simulink model "ModeloManual"  (R2022a)
settings: Solver=VariableStepAuto  StartTime=0.0  StopTime=10  RelTol=1e-3
values from neighbouring files (symbols this model uses):
  a = 0.2    [Data.m]
  alturaobst = 0.9    [Data.m]
  b = 0.542    [Data.m]
  M = [x_new y_new]    [Data.m]
  M_chasis = 3    [Data.m]
  M_rueda = 1    [Data.m]
  M_ruedacontacto = 1    [Data.m]
  N = 4365    [GraficasVelocidades.m]    (also in Prueba_Liapunov.m = length(p_X); WaypointsToTrayectory.m = length(X))
  R = 0.175/2    (= 0.0875)    [Data.m]
  X = M(:,1)    [WaypointsToTrayectory.m]
  x0 = x_ini(1)*factorE    [Data.m]
  x_obj = pos_fin(1)*factorE    [Data.m]
  xobstac = RandomPos(1)    [Data.m]
  Y = M(:, 2)    [WaypointsToTrayectory.m]
  y0 = y_ini(2)*factorE    [Data.m]
  y_obj = pos_fin(2)*factorE    [Data.m]
  yobstac = RandomPos(2)    [Data.m]
  zobstac = RandomPos(3)    [Data.m]
undefined symbols (not defined in the file or in its folder): bloqueobstaculo, Borde11, Borde12, Borde2, Borde3, Borde41, Borde42, Explanada, plano150g1, plano150g2, plano150g3, plano150g4, Plano150mm, plano150mm2irr, Plano45mm, plano45mm2irr, Plano90mm, Rampa, Rampa21, Rampa22, Rampa31, Rampa32, Rampa33, Rampa4, Rampa51, Rampa52, Rampa53, Terreno, Z
libraries: sm_lib x331, nesl_utility x30, fl_lib x3, robotalgslib x1
(part 1 of 8)
settings Model: Creator=User  LastModifiedBy=User
settings ExplorerConfigSet: InternalSimMechanicsExplorerSettings="<ExplorerConfiguration><canonicalview>default</canonicalview><AnimationSetting><BasePlaybackSpeed>1.0</BasePlaybackSpeed><PlaybackSpeedFactor>8.0</PlaybackSpeedFactor></AnimationSetting><TilePanel><TileInfo><Tiles Columns=\"2\" Count=\"2\" Rows=\"1\"><Column Weight=\"0.5166\"/><Column Weight=\"0.4834\"/><Row Weight=\"1\"/><Tile Height=\"1\" Width=\"1\" X=\"0\" Y=\"0\"/><Tile Height=\"1\" Width=\"1\" X=\"1\" Y=\"0\"/></Tiles></TileInfo><SceneInfo><SceneViewer><BGColor><R>0.60000002384185791</R><G>0.60000002384185791</G><B>0.60000002384185791</B></BGColor><Camera><DoPerspective>on</DoPerspective><Position><X>190.872114263138826</X><Y>194.191955454598997</Y><Z>244.498723214842585</Z></Position><Center><X>176.122953180660318</X><Y>239.114971855998164</Y><Z>2.09998758117879447</Z></Center><Up><X>0.0154631214745943289</X><Y>0.983307639935577793</Y><Z>0.181292518098750938</Z></Up><ViewLimDist>1</ViewLimDist><YLim>0.466307658154998583</YLim><XLim>0.450624665167722871</XLim></Camera></SceneViewer><SceneViewer><BGColor><R>0.400000005960464478</R><G>0.800000011920928955</G><B>1</B></BGColor><Camera><DoPerspective>on</DoPerspective><Position><X>214.286586538195536</X><Y>301.219122430627294</Y><Z>1.50750834751243712</Z></Position><Center><X>214.645296115876107</X><Y>302.136282732512313</Y><Z>1.33388686403077461</Z></Center><Up><X>0.0632456935347918969</X><Y>0.16169230597039197</Y><Z>0.984812459526828055</Z></Up><ViewLimDist>1</ViewLimDist><YLim>0.466307658154998583</YLim><XLim>0.421349744924808145</XLim></Camera></SceneViewer></SceneInfo></TilePanel><MechEditorPanel><Cameras><Camera><Id>Camera2</Id><Value><Name>Seguimiento</Name><NativeCamera><PositionTrackingFeature>ROBOT_SS.Ensamble_robot.Chasis.Chasis_Camera_RightB.R</PositionTrackingFeature><CenterTrackingFeature>ROBOT_SS.Ensamble_robot.Chasis.Chasis_Camera_RightB.R</CenterTrackingFeature><UpVectorTrackingFeature>ROBOT_SS.Ensamble_robot.Chasis.Chasis_Camera_RightB.R</UpVectorTrackingFeature><CenterTrackingOrigin>off</CenterTrackingOrigin><CenterTrackingDirection>+X</CenterTrackingDirection><UpVectorTrackingDirection>+Z</UpVectorTrackingDirection></NativeCamera></Value></Camera><Camera><Id>Camera3</Id><Value><Name>Fija</Name><NativeCamera><PositionKeyframeSet><Keyframe><Time>10</Time><Value><X>194.17156367953794</X><Y>236.62255003194693</Y><Z>376.38019149049347</Z></Value></Keyframe></PositionKeyframeSet><CenterKeyframeSet><Keyframe><Time>10</Time><Value><X>194.17156367953794</X><Y>236.62255003194693</Y><Z>15.721481323242188</Z></Value></Keyframe></CenterKeyframeSet><UpVectorKeyframeSet><Keyframe><Time>10</Time><Value><X>0</X><Y>1</Y><Z>-0</Z></Value></Keyframe></UpVectorKeyframeSet></NativeCamera></Value></Camera><Camera><Id>Camera4</Id><Value><Name>lateralVista</Name><NativeCamera><PositionTrackingFeature>ROBOT_SS.Ensamble_robot.Chasis.Chasis_Camera_Rear.R</PositionTrackingFeature><CenterTrackingFeature>ROBOT_SS.Ensamble_robot.Chasis.Chasis_Camera_Rear.R</CenterTrackingFeature><UpVectorTrackingFeature>ROBOT_SS.Ensamble_robot.Chasis.Chasis_Camera_Rear.R</UpVectorTrackingFeature><CenterTrackingOrigin>off</CenterTrackingOrigin><CenterTrackingDirection>-Y</CenterTrackingDirection><UpVectorTrackingDirection>+Z</UpVectorTrackingDirection></NativeCamera></Value></Camera><Camera><Id>Camera5</Id><Value><Name>VistaAsup</Name><NativeCamera><PositionTrackingFeature>ROBOT_SS.Ensamble_robot.Chasis.Chasis_Camera_RightA.R</PositionTrackingFeature><CenterTrackingFeature>ROBOT_SS.Ensamble_robot.Chasis.Chasis_Camera_RightA.R</CenterTrackingFeature><UpVectorTrackingFeature>ROBOT_SS.Ensamble_robot.Chasis.Chasis_Camera_RightA.R</UpVectorTrackingFeature><CenterTrackingOrigin>off</CenterTrackingOrigin><CenterTrackingDirection>+X</CenterTrackingDirection><UpVectorTrackingDirection>+Z</UpVectorTrackingDirection></NativeCamera></Value></Camera><Camera><Id>Camera6</Id><Value><Name>VistaB</Name><NativeCamera><PositionTrackingFeature>ROBOT_SS.Ensamble_robot.Chasis.Chasis_Camera_RightB.R</PositionTrackingFeature><CenterTrackingFeature>ROBOT_SS.Ensamble_robot.Chasis.Chasis_Camera_RightB.R</CenterTrackingFeature><UpVectorTrackingFeature>ROBOT_SS.Ensamble_robot.Chasis.Chasis_Camera_RightB.R</UpVectorTrackingFeature><CenterTrackingOrigin>off</CenterTrackingOrigin><CenterTrackingDirection>+X</CenterTrackingDirection><UpVectorTrackingDirection>+Z</UpVectorTrackingDirection></NativeCamera></Value></Camera><Camera><Id>Camera7</Id><Value><Name>Top</Name><NativeCamera><PositionKeyframeSet><Keyframe><Time>0</Time><Value><X>190.87211426313883</X><Y>194.191955454599</Y><Z>244.49872321484258</Z></Value></Keyframe></PositionKeyframeSet><CenterKeyframeSet><Keyframe><Time>0</Time><Value><X>176.12295318066032</X><Y>239.11497185599816</Y><Z>2.0999875811787945</Z></Value></Keyframe></CenterKeyframeSet><UpVectorKeyframeSet><Keyframe><Time>0</Time><Value><X>0.015463121474594329</X><Y>0.98330763993557779</Y><Z>0.18129251809875094</Z></Value></Keyframe></UpVectorKeyframeSet></NativeCamera></Value></Camera></Cameras><GfxPanelCameraMap><MapElement CameraMLId=\"Camera7\" GfxPanelIndex=\"0\"/><MapElement CameraMLId=\"Camera5\" GfxPanelIndex=\"1\"/></GfxPanelCameraMap><VideoCreator><PlaybackSpeedRatio>4.0</PlaybackSpeedRatio><FrameRate>60</FrameRate><VideoFormat>MPEG-4</VideoFormat><FrameSize>auto</FrameSize></VideoCreator></MechEditorPanel></ExplorerConfiguration>"

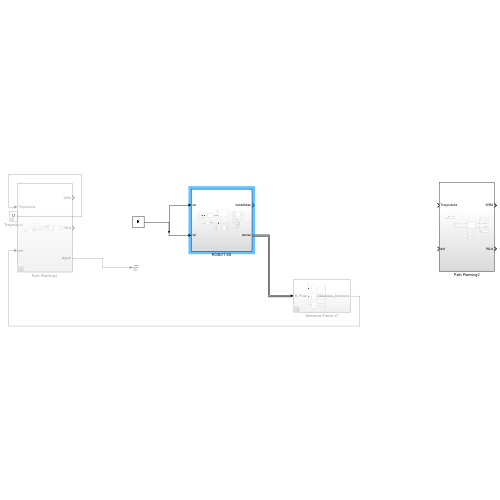
[thumbnail: Simulink's stored preview of the top-level diagram]
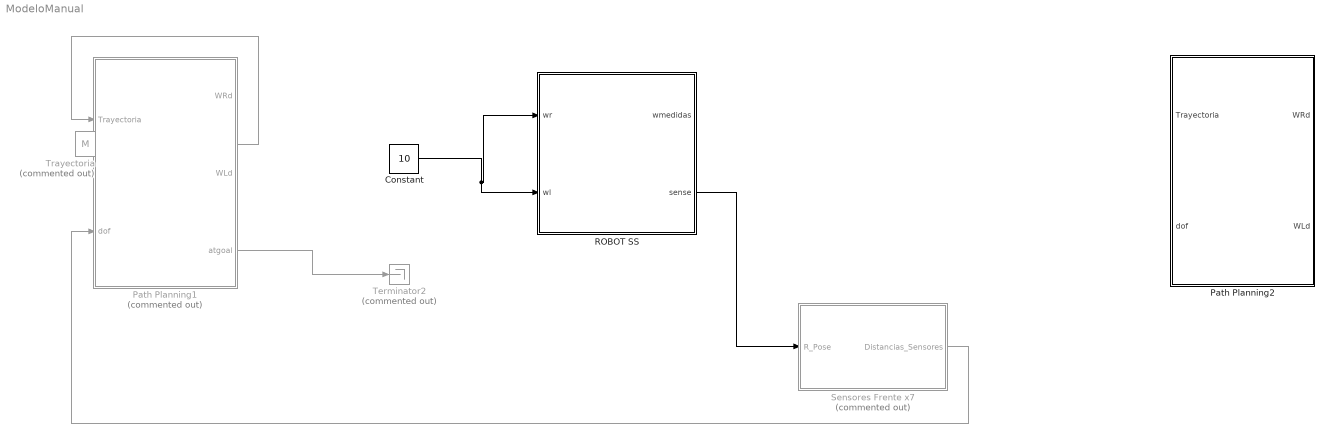
== system ModeloManual ==
  Constant : Constant  Value=10
  Path Planning1 : Subsystem  Commented=on
  Path Planning2 : Subsystem
  ROBOT SS : Subsystem
  Sensores Frente x7 : Subsystem  Commented=on
  Terminator2 : Terminator  Commented=on
  Trayectoria : Constant  Commented=on  Value=M
  wires:
  Path Planning1/3(atgoal) -> Terminator2/1
  Trayectoria/1 -> Path Planning1/1(Trayectoria)
  ROBOT SS/2(sense) -> Sensores Frente x7/1(R_Pose)
  Constant/1 -> ROBOT SS/2(wl), ROBOT SS/1(wr)
  Sensores Frente x7/1(Distancias_Sensores) -> Path Planning1/2(dof)

== system ModeloManual/Path Planning1 ==
  note: Des Wspeed
  Trayectoria : Inport
  In Bus Element : Inport  Port=2  PortName=dof  Element=Pose
  Clock : Clock
  Constant : Constant  Value=0.5
  Kinematics1 : Subsystem
  Pure  Pursuit2 : robotalgslib/Pure Pursuit  DesiredLinearVelocity=1.38  MaxAngularVelocity=pi  LookaheadDistance=0.05  TargetDirPort=on  SimulateUsing=Interpreted execution
  Subsystem1 : Subsystem
  Terminator : Terminator
  Terminator1 : Terminator
  To Workspace : ToWorkspace  VariableName=RobotPose  SampleTime=-1
  Trapezoidal Vel Profile : MATLAB Function  TreatAsAtomicUnit=on
  hold : Subsystem
  t1 : Constant
  WRd : Outport
  WLd : Outport  Port=2
  atgoal : Outport  Port=3
  wires:
  Pure  Pursuit2/1 -> Trapezoidal Vel Profile/1(linVel), Subsystem1/1(linearV)
  Constant/1 -> Trapezoidal Vel Profile/4(accel)
  Clock/1 -> Trapezoidal Vel Profile/2(t)
  Kinematics1/1(WRd) -> WRd/1
  Pure  Pursuit2/2 -> Kinematics1/2(w)
  Trapezoidal Vel Profile/1(lin_Vel_out) -> Kinematics1/1(v)
  t1/1 -> Trapezoidal Vel Profile/3(t1)
  hold/1(deaccelStartTime) -> Trapezoidal Vel Profile/5(deaccelStartTime)
  Trayectoria/1 -> Pure  Pursuit2/2
  Subsystem1/2(atgoal) -> atgoal/1
  Subsystem1/1(deAcc) -> hold/1(deAcc)
  Kinematics1/2(WLd) -> WLd/1
  In Bus Element/1 -> Subsystem1/2(Pose), To Workspace/1, Pure  Pursuit2/1
  Pure  Pursuit2/3 -> Terminator/1
  Kinematics1/3(Pose) -> Terminator1/1

== system ModeloManual/Path Planning2 ==
  Trayectoria : Inport
  In Bus Element : Inport  Port=2  PortName=dof  Element=Pose
  Constant : Constant  Value=1.38
  Constant1 : Constant  Value=0
  Display{,1..3} (4 alike) : Display
  Kinematics1 : Subsystem
  Waypoint Tracking Logic : Stateflow chart  Commented=on  TreatAsAtomicUnit=on
  WRd : Outport
  WLd : Outport  Port=2
  wires:
  Constant1/1 -> Kinematics1/2(w)
  Constant/1 -> Kinematics1/1(v)
  Trayectoria/1 -> Waypoint Tracking Logic/2(waypoints)
  In Bus Element/1 -> Waypoint Tracking Logic/1(pose)
  Kinematics1/2(WLd) -> WLd/1, Display3/1
  Kinematics1/1(WRd) -> Display1/1, WRd/1

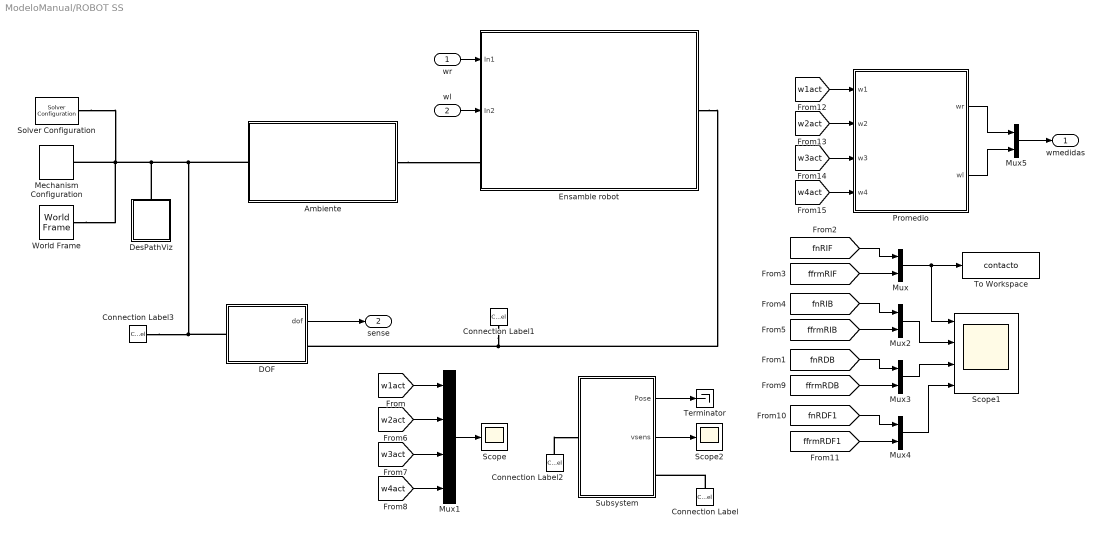
== system ModeloManual/ROBOT SS ==
  wr : Inport
  wl : Inport  Port=2
  Ambiente : Subsystem
  Connection Label : ConnectionLabel  Label=Ref
  Connection Label1 : ConnectionLabel  Label=Ref
  Connection Label2 : ConnectionLabel  Label=B
  Connection Label3 : ConnectionLabel  Label=B
  DOF : Subsystem
  DesPathViz : Subsystem
  Ensamble robot : Subsystem
  Mechanism Configuration : sm_lib/Utilities/Mechanism Configuration  UniformGravity=Constant  GravityVector=[0 0 -9.80665]  GravityUnits=m/s^2  LinearizationDelta=0.001  JointModeTransitionNonlinearIterations=2
  Mux{,2..5} (5 alike) : Mux  Inputs=2
  Mux1 : Mux
  Promedio : MATLAB Function  TreatAsAtomicUnit=on
  Scope : Scope
  Scope1 : Scope  NumInputPorts=4
  Scope2 : Scope
  Solver Configuration : nesl_utility/Solver Configuration  PhysicalDomain=network_engine_domain  SubClassName=solver  LeftPortType=input  RightPortType=generic  Tones=[]  Harmonics=[]  SimulateNoise=off  Profile=off  UseLocalSampling=off  EnableSwitchedLinearOptims=on  FrequencyDomain=off  UseCCode=off  RelTol=0.001  AbsTol=0.001  MinStep=1e-09  ToWorkspace=off  RevertToSquareIcSolve=off  NumHomotopyIterations=100  PhasorMode=off  PhasorModeNumHarmonics=1  IndexReductionMethod=DerivativeReplacement  DoDC=off  ResidualTolerance=1e-09  UseLocalSolver=off  LocalSolverChoice=NE_BACKWARD_EULER_ADVANCER  LocalSolverSampleTime=0.001  DoFixedCost=off  MaxNonlinIter=3  MaxModeIter=2  ComputeImpulses=off  ImpulseIterations=2  LinearAlgebra=auto  LinearAlgebraNumThread=0  EquationFormulation=NE_TIME_EF  DelaysMemoryBudget=1024  AutomaticFiltering=on  FilteringTimeConstant=0.001  PartitionStorageMethod=AS_NEEDED  PartitionMemoryBudget=1024  PartitionMethod=ROBUST
      settings: SourceProductBaseCode=SS,PW,VE
  Subsystem : Subsystem
  Terminator : Terminator
  To Workspace : ToWorkspace  VariableName=contacto  SaveFormat=Timeseries  SampleTime=-1
  World Frame : sm_lib/Frames and Transforms/World Frame
  wmedidas : Outport
  sense : Outport  Port=2
  wires:
  [w3act] -> Mux1/3
  [w1act] -> Mux1/1
  Mux1/1 -> Scope/1
  [w2act] -> Mux1/2
  [w4act] -> Mux1/4
  [ffrmRDB] -> Mux3/2
  Mux/1 -> Scope1/1, To Workspace/1
  [ffrmRIF] -> Mux/2
  [ffrmRIB] -> Mux2/2
  [fnRDB] -> Mux3/1
  Mux3/1 -> Scope1/3
  [fnRIF] -> Mux/1
  Mux2/1 -> Scope1/2
  Mux4/1 -> Scope1/4
  [fnRDF1] -> Mux4/1
  [fnRIB] -> Mux2/1
  [ffrmRDF1] -> Mux4/2
  Mux5/1 -> wmedidas/1
  [w3act] -> Promedio/3(w3)
  [w4act] -> Promedio/4(w4)
  [w1act] -> Promedio/1(w1)
  Promedio/2(wl) -> Mux5/2
  [w2act] -> Promedio/2(w2)
  Promedio/1(wr) -> Mux5/1
  DOF/1(dof) -> sense/1
  Subsystem/2(vsens) -> Scope2/1
  Subsystem/1(Pose) -> Terminator/1
  wr/1 -> Ensamble robot/1(In1)
  wl/1 -> Ensamble robot/2(In2)
  connections:
  Connection Label/LConn1 -- Subsystem/RConn1
  Connection Label2/LConn1 -- Subsystem/LConn1
  Ensamble robot/RConn1 -- DOF/RConn1 -- Connection Label1/LConn1
  Ambiente/RConn1 -- Ensamble robot/LConn1
  DOF/LConn1 -- Ambiente/LConn1 -- Solver Configuration/RConn1 -- Mechanism Configuration/RConn1 -- World Frame/RConn1 -- DesPathViz/LConn1 -- Connection Label3/LConn1

== system ModeloManual/Sensores Frente x7 ==
  R_Pose : Inport
  Mux : Mux  Inputs=7
  Percepción_Central : Subsystem
  Percepción_Derecha : Subsystem
  Percepción_Izquierda : Subsystem
  Distancias_Sensores : Outport
  wires:
  Percepción_Derecha/2(d_7) -> Mux/7
  Percepción_Central/2(d_4) -> Mux/4
  Percepción_Derecha/1(d_6) -> Mux/6
  Percepción_Izquierda/2(d_2) -> Mux/2
  Percepción_Central/1(d_3) -> Mux/3
  R_Pose/1 -> Percepción_Izquierda/1(R_Pose), Percepción_Central/1(R_Pose), Percepción_Derecha/1(R_Pose)
  Percepción_Izquierda/1(d_1) -> Mux/1
  Percepción_Central/3(d_5) -> Mux/5
  Mux/1 -> Distancias_Sensores/1

== system ModeloManual/Path Planning1/Kinematics1 ==
  v : Inport
  w : Inport  Port=2
  Direct-Kinematics : Subsystem
  Inverse-Kinematics : Subsystem
  Scope1 : Scope  NumInputPorts=2
  WRd : Outport
  WLd : Outport  Port=2
  Pose : Outport  Port=3
  wires:
  Direct-Kinematics/1(Pose) -> Pose/1
  Inverse-Kinematics/1(wL) -> WLd/1, Direct-Kinematics/1(wl), Scope1/1
  Inverse-Kinematics/2(wR) -> WRd/1, Direct-Kinematics/2(wr), Scope1/2
  w/1 -> Direct-Kinematics/3(w), Inverse-Kinematics/2(w)
  v/1 -> Inverse-Kinematics/1(v)

== system ModeloManual/Path Planning1/Subsystem1 ==
  linearV : Inport
  Pose : Inport  Port=2
  Add : Sum
  Constant : Constant  Value=2* 0.5
  Constant1 : Constant  Value=0.25
  Gain : Gain
  GreaterThan : RelationalOperator  Operator=>  OutDataTypeStr=boolean  RndMeth=Simplest  InputSameDT=off
  GreaterThan1 : RelationalOperator  Operator=>  OutDataTypeStr=boolean  RndMeth=Simplest  InputSameDT=off
  NOT : Logic  Operator=NOT  IconShape=distinctive  AllPortsSameDT=off  OutDataTypeStr=boolean
  Product : Product  Inputs=*/
  Square : Math  Operator=square
  Unit Delay : UnitDelay  SampleTime=-1  HasFrameUpgradeWarning=on
  check-goal : Subsystem
  deAcc : Outport
  atgoal : Outport  Port=2
  wires:
  check-goal/1(distanceGoal) -> GreaterThan/1, GreaterThan1/1
  Constant/1 -> Product/2
  Constant1/1 -> GreaterThan1/2, Gain/1
  Add/1 -> GreaterThan/2
  Product/1 -> Add/1
  GreaterThan1/1 -> NOT/1
  Square/1 -> Product/1
  GreaterThan/1 -> deAcc/1
  NOT/1 -> Unit Delay/1
  Pose/1 -> check-goal/1(Pose)
  Unit Delay/1 -> atgoal/1
  linearV/1 -> Square/1
  Gain/1 -> Add/2

== system ModeloManual/Path Planning1/hold ==
  deAcc : Inport
  Constant9 : Constant  Value=inf
  NOT1 : Logic  Operator=NOT  IconShape=distinctive  AllPortsSameDT=off  OutDataTypeStr=boolean
  StopTime : Subsystem
  Switch3 : Switch  Criteria=u2 > Threshold  SaturateOnIntegerOverflow=off  InputSameDT=off
  Unit Delay1 : UnitDelay  SampleTime=-1  HasFrameUpgradeWarning=on
  deaccelStartTime : Outport
  wires:
  Unit Delay1/1 -> Switch3/2
  StopTime/1(DeAccelTime) -> Switch3/1
  Switch3/1 -> deaccelStartTime/1
  NOT1/1 -> StopTime/1(Enable), Unit Delay1/1
  Constant9/1 -> Switch3/3
  deAcc/1 -> NOT1/1

== system ModeloManual/Path Planning2/Kinematics1 ==
  v : Inport
  w : Inport  Port=2
  Inverse-Kinematics : Subsystem
  Scope1 : Scope  NumInputPorts=2
  WRd : Outport
  WLd : Outport  Port=2
  wires:
  v/1 -> Inverse-Kinematics/1(v)
  w/1 -> Inverse-Kinematics/2(w)
  Inverse-Kinematics/2(wR) -> Scope1/2, WRd/1
  Inverse-Kinematics/1(wL) -> Scope1/1, WLd/1

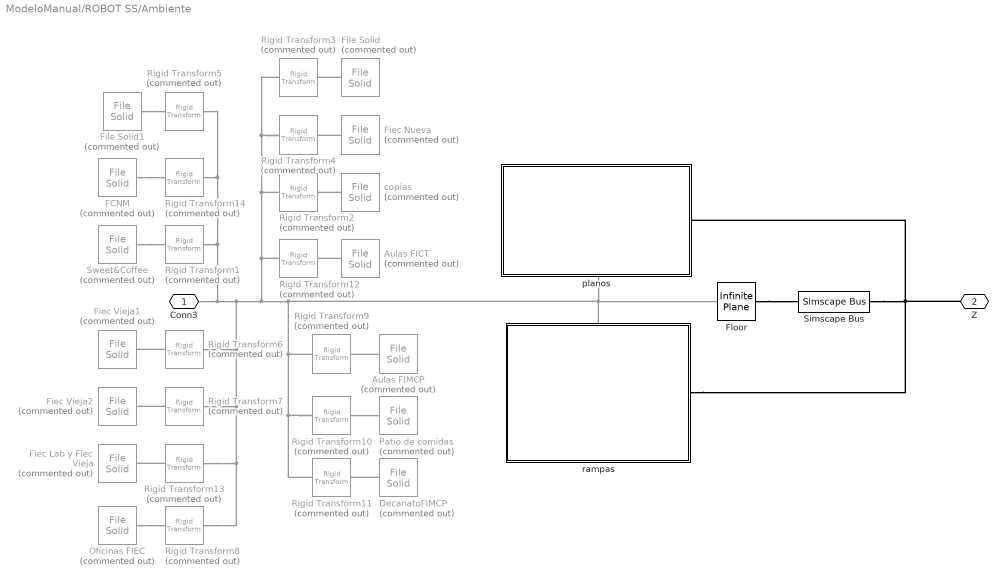
== system ModeloManual/ROBOT SS/Ambiente ==
  Aulas FICT : sm_lib/Body Elements/File Solid  Commented=on  ExtGeomFileName=Edificios\FICT.stl  UnitType=Custom  ExtGeomFileUnits=m  StepReaderType=HEX  ExportConvexHullGeometry=off  InertiaType=PointMass  Mass=1000  MassUnits=kg  CenterOfMass=[0 0 0]  CenterOfMassUnits=m  MomentsOfInertia=[1 1 1]  MomentsOfInertiaUnits=kg*m^2  ProductsOfInertia=[0 0 0]  ProductsOfInertiaUnits=kg*m^2  BasedOnType=DensityFromFile  Density=1000  DensityUnits=kg/m^3  DoExposeReferenceFrame=on  SerializedFrames=<Frames/>  GraphicType=FromGeometry  MarkerShape=Sphere  MarkerSize=10  GraphicVisPropType=SimpleVisualProperties  GraphicDiffuseColor=[0.2 0.4 0.0]  GraphicSpecularColor=[0.5 0.5 0.5 1.0]  GraphicAmbientColor=[0.15 0.15 0.15 1.0]  GraphicEmissiveColor=[0.0 0.0 0.0 1.0]  GraphicShininess=75  GraphicOpacity=1.0
  Aulas FIMCP : sm_lib/Body Elements/File Solid  Commented=on  ExtGeomFileName=Edificios\AulasFIMCP.stl  UnitType=Custom  ExtGeomFileUnits=m  StepReaderType=HEX  ExportConvexHullGeometry=off  InertiaType=PointMass  Mass=1000  MassUnits=kg  CenterOfMass=[0 0 0]  CenterOfMassUnits=m  MomentsOfInertia=[1 1 1]  MomentsOfInertiaUnits=kg*m^2  ProductsOfInertia=[0 0 0]  ProductsOfInertiaUnits=kg*m^2  BasedOnType=DensityFromFile  Density=1000  DensityUnits=kg/m^3  DoExposeReferenceFrame=on  SerializedFrames=<Frames/>  GraphicType=FromGeometry  MarkerShape=Sphere  MarkerSize=10  GraphicVisPropType=SimpleVisualProperties  GraphicDiffuseColor=[0.0 0.0 1.0]  GraphicSpecularColor=[0.5 0.5 0.5 1.0]  GraphicAmbientColor=[0.15 0.15 0.15 1.0]  GraphicEmissiveColor=[0.0 0.0 0.0 1.0]  GraphicShininess=75  GraphicOpacity=1.0
  DecanatoFIMCP : sm_lib/Body Elements/File Solid  Commented=on  ExtGeomFileName=Edificios\LDecanatoFIMCP.stl  UnitType=Custom  ExtGeomFileUnits=m  StepReaderType=HEX  ExportConvexHullGeometry=off  InertiaType=PointMass  Mass=1000  MassUnits=kg  CenterOfMass=[0 0 0]  CenterOfMassUnits=m  MomentsOfInertia=[1 1 1]  MomentsOfInertiaUnits=kg*m^2  ProductsOfInertia=[0 0 0]  ProductsOfInertiaUnits=kg*m^2  BasedOnType=DensityFromFile  Density=1000  DensityUnits=kg/m^3  DoExposeReferenceFrame=on  SerializedFrames=<Frames/>  GraphicType=FromGeometry  MarkerShape=Sphere  MarkerSize=10  GraphicVisPropType=SimpleVisualProperties  GraphicDiffuseColor=[0.0 0.0 1.0]  GraphicSpecularColor=[0.5 0.5 0.5 1.0]  GraphicAmbientColor=[0.15 0.15 0.15 1.0]  GraphicEmissiveColor=[0.0 0.0 0.0 1.0]  GraphicShininess=75  GraphicOpacity=1.0
  FCNM : sm_lib/Body Elements/File Solid  Commented=on  ExtGeomFileName=Edificios\FCNM.stl  UnitType=Custom  ExtGeomFileUnits=m  StepReaderType=HEX  ExportConvexHullGeometry=off  InertiaType=PointMass  Mass=100  MassUnits=kg  CenterOfMass=[0 0 0]  CenterOfMassUnits=m  MomentsOfInertia=[1 1 1]  MomentsOfInertiaUnits=kg*m^2  ProductsOfInertia=[0 0 0]  ProductsOfInertiaUnits=kg*m^2  BasedOnType=DensityFromFile  Density=1000  DensityUnits=kg/m^3  DoExposeReferenceFrame=on  SerializedFrames=<Frames/>  GraphicType=FromGeometry  MarkerShape=Sphere  MarkerSize=10  GraphicVisPropType=SimpleVisualProperties  GraphicDiffuseColor=[0.4 0.0 0.8]  GraphicSpecularColor=[0.5 0.5 0.5 1.0]  GraphicAmbientColor=[0.15 0.15 0.15 1.0]  GraphicEmissiveColor=[0.0 0.0 0.0 1.0]  GraphicShininess=75  GraphicOpacity=1.0
  Fiec Lab y Fiec Vieja : sm_lib/Body Elements/File Solid  Commented=on  ExtGeomFileName=Edificios\LabFiec_FiecVieja.stl  UnitType=Custom  ExtGeomFileUnits=m  StepReaderType=HEX  ExportConvexHullGeometry=off  InertiaType=PointMass  Mass=100  MassUnits=kg  CenterOfMass=[0 0 0]  CenterOfMassUnits=m  MomentsOfInertia=[1 1 1]  MomentsOfInertiaUnits=kg*m^2  ProductsOfInertia=[0 0 0]  ProductsOfInertiaUnits=kg*m^2  BasedOnType=DensityFromFile  Density=1000  DensityUnits=kg/m^3  DoExposeReferenceFrame=on  SerializedFrames=<Frames/>  GraphicType=FromGeometry  MarkerShape=Sphere  MarkerSize=10  GraphicVisPropType=SimpleVisualProperties  GraphicDiffuseColor=[0.8 0.2 0.0]  GraphicSpecularColor=[0.5 0.5 0.5 1.0]  GraphicAmbientColor=[0.15 0.15 0.15 1.0]  GraphicEmissiveColor=[0.0 0.0 0.0 1.0]  GraphicShininess=75  GraphicOpacity=1.0
  Fiec Nueva : sm_lib/Body Elements/File Solid  Commented=on  ExtGeomFileName=Edificios\fiecNueva.stl  UnitType=Custom  ExtGeomFileUnits=m  StepReaderType=HEX  ExportConvexHullGeometry=off  InertiaType=PointMass  Mass=1000  MassUnits=kg  CenterOfMass=[0 0 0]  CenterOfMassUnits=m  MomentsOfInertia=[1 1 1]  MomentsOfInertiaUnits=kg*m^2  ProductsOfInertia=[0 0 0]  ProductsOfInertiaUnits=kg*m^2  BasedOnType=DensityFromFile  Density=1000  DensityUnits=kg/m^3  DoExposeReferenceFrame=on  SerializedFrames=<Frames/>  GraphicType=FromGeometry  MarkerShape=Sphere  MarkerSize=10  GraphicVisPropType=SimpleVisualProperties  GraphicDiffuseColor=[0.8 0.2 0.0]  GraphicSpecularColor=[0.5 0.5 0.5 1.0]  GraphicAmbientColor=[0.15 0.15 0.15 1.0]  GraphicEmissiveColor=[0.0 0.0 0.0 1.0]  GraphicShininess=75  GraphicOpacity=1.0
  Fiec Vieja1 : sm_lib/Body Elements/File Solid  Commented=on  ExtGeomFileName=Edificios\fiecVieja.stl  UnitType=Custom  ExtGeomFileUnits=m  StepReaderType=HEX  ExportConvexHullGeometry=off  InertiaType=PointMass  Mass=100  MassUnits=kg  CenterOfMass=[0 0 0]  CenterOfMassUnits=m  MomentsOfInertia=[1 1 1]  MomentsOfInertiaUnits=kg*m^2  ProductsOfInertia=[0 0 0]  ProductsOfInertiaUnits=kg*m^2  BasedOnType=DensityFromFile  Density=1000  DensityUnits=kg/m^3  DoExposeReferenceFrame=on  SerializedFrames=<Frames/>  GraphicType=FromGeometry  MarkerShape=Sphere  MarkerSize=10  GraphicVisPropType=SimpleVisualProperties  GraphicDiffuseColor=[0.8 0.2 0.0]  GraphicSpecularColor=[0.5 0.5 0.5 1.0]  GraphicAmbientColor=[0.15 0.15 0.15 1.0]  GraphicEmissiveColor=[0.0 0.0 0.0 1.0]  GraphicShininess=75  GraphicOpacity=1.0
  Fiec Vieja2 : sm_lib/Body Elements/File Solid  Commented=on  ExtGeomFileName=Edificios\fiecVieja.stl  UnitType=Custom  ExtGeomFileUnits=m  StepReaderType=HEX  ExportConvexHullGeometry=off  InertiaType=PointMass  Mass=100  MassUnits=kg  CenterOfMass=[0 0 0]  CenterOfMassUnits=m  MomentsOfInertia=[1 1 1]  MomentsOfInertiaUnits=kg*m^2  ProductsOfInertia=[0 0 0]  ProductsOfInertiaUnits=kg*m^2  BasedOnType=DensityFromFile  Density=1000  DensityUnits=kg/m^3  DoExposeReferenceFrame=on  SerializedFrames=<Frames/>  GraphicType=FromGeometry  MarkerShape=Sphere  MarkerSize=10  GraphicVisPropType=SimpleVisualProperties  GraphicDiffuseColor=[0.8 0.2 0.0]  GraphicSpecularColor=[0.5 0.5 0.5 1.0]  GraphicAmbientColor=[0.15 0.15 0.15 1.0]  GraphicEmissiveColor=[0.0 0.0 0.0 1.0]  GraphicShininess=75  GraphicOpacity=1.0
  File Solid : sm_lib/Body Elements/File Solid  Commented=on  ExtGeomFileName=Edificios\Tree2.stl  UnitType=Custom  ExtGeomFileUnits=m  StepReaderType=HEX  ExportConvexHullGeometry=off  InertiaType=CalculateFromGeometry  Mass=1  MassUnits=kg  CenterOfMass=[0 0 0]  CenterOfMassUnits=m  MomentsOfInertia=[1 1 1]  MomentsOfInertiaUnits=kg*m^2  ProductsOfInertia=[0 0 0]  ProductsOfInertiaUnits=kg*m^2  BasedOnType=Density  Density=1000  DensityUnits=kg/m^3  DoExposeReferenceFrame=on  SerializedFrames=<Frames/>  GraphicType=FromGeometry  MarkerShape=Sphere  MarkerSize=10  GraphicVisPropType=SimpleVisualProperties  GraphicDiffuseColor=[0.6 0.8 0.0]  GraphicSpecularColor=[0.5 0.5 0.5 1.0]  GraphicAmbientColor=[0.15 0.15 0.15 1.0]  GraphicEmissiveColor=[0.0 0.0 0.0 1.0]  GraphicShininess=75  GraphicOpacity=1.0
  File Solid1 : sm_lib/Body Elements/File Solid  Commented=on  ExtGeomFileName=Edificios\Tree2.stl  UnitType=Custom  ExtGeomFileUnits=m  StepReaderType=HEX  ExportConvexHullGeometry=off  InertiaType=CalculateFromGeometry  Mass=1  MassUnits=kg  CenterOfMass=[0 0 0]  CenterOfMassUnits=m  MomentsOfInertia=[1 1 1]  MomentsOfInertiaUnits=kg*m^2  ProductsOfInertia=[0 0 0]  ProductsOfInertiaUnits=kg*m^2  BasedOnType=Density  Density=1000  DensityUnits=kg/m^3  DoExposeReferenceFrame=on  SerializedFrames=<Frames/>  GraphicType=FromGeometry  MarkerShape=Sphere  MarkerSize=10  GraphicVisPropType=SimpleVisualProperties  GraphicDiffuseColor=[0.6 0.8 0.0]  GraphicSpecularColor=[0.5 0.5 0.5 1.0]  GraphicAmbientColor=[0.15 0.15 0.15 1.0]  GraphicEmissiveColor=[0.0 0.0 0.0 1.0]  GraphicShininess=75  GraphicOpacity=1.0
  Floor : sm_lib/Curves and Surfaces/Infinite Plane  GraphicType=Rectangle  GraphicPlaneWidth=1600  GraphicPlaneWidthUnits=m  GraphicPlaneHeight=1000  GraphicPlaneHeightUnits=m  GraphicVisPropType=SimpleVisualProperties  GraphicDiffuseColor=[0.8 0.8 0.8]  GraphicOpacity=1  GraphicSpecularColor=[0.5 0.5 0.5 1.0]  GraphicAmbientColor=[0.15 0.15 0.15 1.0]  GraphicEmissiveColor=[0.0 0.0 0.0 1.0]  GraphicShininess=75
  Oficinas FIEC : sm_lib/Body Elements/File Solid  Commented=on  ExtGeomFileName=Edificios\oficinaFiec.stl  UnitType=Custom  ExtGeomFileUnits=m  StepReaderType=HEX  ExportConvexHullGeometry=off  InertiaType=PointMass  Mass=100  MassUnits=kg  CenterOfMass=[0 0 0]  CenterOfMassUnits=m  MomentsOfInertia=[1 1 1]  MomentsOfInertiaUnits=kg*m^2  ProductsOfInertia=[0 0 0]  ProductsOfInertiaUnits=kg*m^2  BasedOnType=DensityFromFile  Density=1000  DensityUnits=kg/m^3  DoExposeReferenceFrame=on  SerializedFrames=<Frames/>  GraphicType=FromGeometry  MarkerShape=Sphere  MarkerSize=10  GraphicVisPropType=SimpleVisualProperties  GraphicDiffuseColor=[0.8 0.2 0]  GraphicSpecularColor=[0.5 0.5 0.5 1.0]  GraphicAmbientColor=[0.15 0.15 0.15 1.0]  GraphicEmissiveColor=[0.0 0.0 0.0 1.0]  GraphicShininess=75  GraphicOpacity=1.0
  Patio de comidas : sm_lib/Body Elements/File Solid  Commented=on  ExtGeomFileName=Edificios\patiodecomida.stl  UnitType=Custom  ExtGeomFileUnits=m  StepReaderType=HEX  ExportConvexHullGeometry=off  InertiaType=PointMass  Mass=1000  MassUnits=kg  CenterOfMass=[0 0 0]  CenterOfMassUnits=m  MomentsOfInertia=[1 1 1]  MomentsOfInertiaUnits=kg*m^2  ProductsOfInertia=[0 0 0]  ProductsOfInertiaUnits=kg*m^2  BasedOnType=DensityFromFile  Density=1000  DensityUnits=kg/m^3  DoExposeReferenceFrame=on  SerializedFrames=<Frames/>  GraphicType=FromGeometry  MarkerShape=Sphere  MarkerSize=10  GraphicVisPropType=SimpleVisualProperties  GraphicDiffuseColor=[1.0 1.0 0.0]  GraphicSpecularColor=[0.5 0.5 0.5 1.0]  GraphicAmbientColor=[0.15 0.15 0.15 1.0]  GraphicEmissiveColor=[0.0 0.0 0.0 1.0]  GraphicShininess=75  GraphicOpacity=1.0
  Rigid Transform1 : sm_lib/Frames and Transforms/Rigid Transform  Commented=on  TranslationMethod=Cartesian  TranslationStandardOffset=0  TranslationLengthUnit=m  TranslationStandardAxis=+Z  TranslationCartesianOffset=[-160 -250 0]  TranslationROffset=0  TranslationROffsetUnits=m  TranslationZOffset=0  TranslationZOffsetUnits=m  TranslationThetaOffset=0  TranslationThetaOffsetUnits=deg  RotationMethod=StandardAxis  RotationAngleUnits=deg  RotationStandardAxis=+Z  RotationAngle=0  RotationArbitraryAxis=[0 0 1]  FollAlignAxisA=+X  BaseAlignAxisA=+Y  FollAlignAxisB=+Y  BaseAlignAxisB=+Z  RotationSequenceAxes=FollowerAxes  RotationSequence=XYX  RotationSequenceAngles=[0 0 0]  RotationSequenceAnglesUnits=deg  RotationMatrix=[1 0 0; 0 1 0; 0 0 1]
  Rigid Transform10 : sm_lib/Frames and Transforms/Rigid Transform  Commented=on  TranslationMethod=Cartesian  TranslationStandardOffset=0  TranslationLengthUnit=m  TranslationStandardAxis=+Z  TranslationCartesianOffset=[-160 -249.5 0]  TranslationROffset=0  TranslationROffsetUnits=m  TranslationZOffset=0  TranslationZOffsetUnits=m  TranslationThetaOffset=0  TranslationThetaOffsetUnits=deg  RotationMethod=StandardAxis  RotationAngleUnits=deg  RotationStandardAxis=+Z  RotationAngle=0  RotationArbitraryAxis=[0 0 1]  FollAlignAxisA=+X  BaseAlignAxisA=+Y  FollAlignAxisB=+Y  BaseAlignAxisB=+Z  RotationSequenceAxes=FollowerAxes  RotationSequence=XYX  RotationSequenceAngles=[0 0 0]  RotationSequenceAnglesUnits=deg  RotationMatrix=[1 0 0; 0 1 0; 0 0 1]
  Rigid Transform11 : sm_lib/Frames and Transforms/Rigid Transform  Commented=on  TranslationMethod=Cartesian  TranslationStandardOffset=0  TranslationLengthUnit=m  TranslationStandardAxis=+Z  TranslationCartesianOffset=[-215 -240 0]  TranslationROffset=0  TranslationROffsetUnits=m  TranslationZOffset=0  TranslationZOffsetUnits=m  TranslationThetaOffset=0  TranslationThetaOffsetUnits=deg  RotationMethod=StandardAxis  RotationAngleUnits=deg  RotationStandardAxis=+Z  RotationAngle=0  RotationArbitraryAxis=[0 0 1]  FollAlignAxisA=+X  BaseAlignAxisA=+Y  FollAlignAxisB=+Y  BaseAlignAxisB=+Z  RotationSequenceAxes=FollowerAxes  RotationSequence=XYX  RotationSequenceAngles=[0 0 0]  RotationSequenceAnglesUnits=deg  RotationMatrix=[1 0 0; 0 1 0; 0 0 1]
  Rigid Transform12 : sm_lib/Frames and Transforms/Rigid Transform  Commented=on  TranslationMethod=Cartesian  TranslationStandardOffset=0  TranslationLengthUnit=m  TranslationStandardAxis=+Z  TranslationCartesianOffset=[-192 -178 0]  TranslationROffset=0  TranslationROffsetUnits=m  TranslationZOffset=0  TranslationZOffsetUnits=m  TranslationThetaOffset=0  TranslationThetaOffsetUnits=deg  RotationMethod=StandardAxis  RotationAngleUnits=deg  RotationStandardAxis=+Z  RotationAngle=0  RotationArbitraryAxis=[0 0 1]  FollAlignAxisA=+X  BaseAlignAxisA=+Y  FollAlignAxisB=+Y  BaseAlignAxisB=+Z  RotationSequenceAxes=FollowerAxes  RotationSequence=XYX  RotationSequenceAngles=[0 0 0]  RotationSequenceAnglesUnits=deg  RotationMatrix=[1 0 0; 0 1 0; 0 0 1]
  Rigid Transform13 : sm_lib/Frames and Transforms/Rigid Transform  Commented=on  TranslationMethod=Cartesian  TranslationStandardOffset=0  TranslationLengthUnit=m  TranslationStandardAxis=+Z  TranslationCartesianOffset=[-196 -180 0]  TranslationROffset=0  TranslationROffsetUnits=m  TranslationZOffset=0  TranslationZOffsetUnits=m  TranslationThetaOffset=0  TranslationThetaOffsetUnits=deg  RotationMethod=StandardAxis  RotationAngleUnits=deg  RotationStandardAxis=+Z  RotationAngle=0  RotationArbitraryAxis=[0 0 1]  FollAlignAxisA=+X  BaseAlignAxisA=+Y  FollAlignAxisB=+Y  BaseAlignAxisB=+Z  RotationSequenceAxes=FollowerAxes  RotationSequence=XYX  RotationSequenceAngles=[0 0 0]  RotationSequenceAnglesUnits=deg  RotationMatrix=[1 0 0; 0 1 0; 0 0 1]
  Rigid Transform14 : sm_lib/Frames and Transforms/Rigid Transform  Commented=on  TranslationMethod=Cartesian  TranslationStandardOffset=0  TranslationLengthUnit=m  TranslationStandardAxis=+Z  TranslationCartesianOffset=[-192 -180 0]  TranslationROffset=0  TranslationROffsetUnits=m  TranslationZOffset=0  TranslationZOffsetUnits=m  TranslationThetaOffset=0  TranslationThetaOffsetUnits=deg  RotationMethod=StandardAxis  RotationAngleUnits=deg  RotationStandardAxis=+Z  RotationAngle=0  RotationArbitraryAxis=[0 0 1]  FollAlignAxisA=+X  BaseAlignAxisA=+Y  FollAlignAxisB=+Y  BaseAlignAxisB=+Z  RotationSequenceAxes=FollowerAxes  RotationSequence=XYX  RotationSequenceAngles=[0 0 0]  RotationSequenceAnglesUnits=deg  RotationMatrix=[1 0 0; 0 1 0; 0 0 1]
  Rigid Transform2 : sm_lib/Frames and Transforms/Rigid Transform  Commented=on  TranslationMethod=Cartesian  TranslationStandardOffset=0  TranslationLengthUnit=m  TranslationStandardAxis=+Z  TranslationCartesianOffset=[-166 -245 0]  TranslationROffset=0  TranslationROffsetUnits=m  TranslationZOffset=0  TranslationZOffsetUnits=m  TranslationThetaOffset=0  TranslationThetaOffsetUnits=deg  RotationMethod=StandardAxis  RotationAngleUnits=deg  RotationStandardAxis=+Z  RotationAngle=0  RotationArbitraryAxis=[0 0 1]  FollAlignAxisA=+X  BaseAlignAxisA=+Y  FollAlignAxisB=+Y  BaseAlignAxisB=+Z  RotationSequenceAxes=FollowerAxes  RotationSequence=XYX  RotationSequenceAngles=[0 0 0]  RotationSequenceAnglesUnits=deg  RotationMatrix=[1 0 0; 0 1 0; 0 0 1]
  Rigid Transform3 : sm_lib/Frames and Transforms/Rigid Transform  Commented=on  TranslationMethod=Cartesian  TranslationStandardOffset=0  TranslationLengthUnit=m  TranslationStandardAxis=+Z  TranslationCartesianOffset=[-160 -260 0]  TranslationROffset=0  TranslationROffsetUnits=m  TranslationZOffset=0  TranslationZOffsetUnits=m  TranslationThetaOffset=0  TranslationThetaOffsetUnits=deg  RotationMethod=StandardAxis  RotationAngleUnits=deg  RotationStandardAxis=+Z  RotationAngle=0  RotationArbitraryAxis=[0 0 1]  FollAlignAxisA=+X  BaseAlignAxisA=+Y  FollAlignAxisB=+Y  BaseAlignAxisB=+Z  RotationSequenceAxes=FollowerAxes  RotationSequence=XYX  RotationSequenceAngles=[0 0 0]  RotationSequenceAnglesUnits=deg  RotationMatrix=[1 0 0; 0 1 0; 0 0 1]
  Rigid Transform4 : sm_lib/Frames and Transforms/Rigid Transform  Commented=on  TranslationMethod=Cartesian  TranslationStandardOffset=0  TranslationLengthUnit=m  TranslationStandardAxis=+Z  TranslationCartesianOffset=[-175 210 0]  TranslationROffset=0  TranslationROffsetUnits=m  TranslationZOffset=0  TranslationZOffsetUnits=m  TranslationThetaOffset=0  TranslationThetaOffsetUnits=deg  RotationMethod=StandardAxis  RotationAngleUnits=deg  RotationStandardAxis=+Z  RotationAngle=-90.0  RotationArbitraryAxis=[0 0 1]  FollAlignAxisA=+X  BaseAlignAxisA=+Y  FollAlignAxisB=+Y  BaseAlignAxisB=+Z  RotationSequenceAxes=FollowerAxes  RotationSequence=XYX  RotationSequenceAngles=[0 0 0]  RotationSequenceAnglesUnits=deg  RotationMatrix=[1 0 0; 0 1 0; 0 0 1]
  Rigid Transform5 : sm_lib/Frames and Transforms/Rigid Transform  Commented=on  TranslationMethod=Cartesian  TranslationStandardOffset=0  TranslationLengthUnit=m  TranslationStandardAxis=+Z  TranslationCartesianOffset=[-240 -310 0]  TranslationROffset=0  TranslationROffsetUnits=m  TranslationZOffset=0  TranslationZOffsetUnits=m  TranslationThetaOffset=0  TranslationThetaOffsetUnits=deg  RotationMethod=StandardAxis  RotationAngleUnits=deg  RotationStandardAxis=+Z  RotationAngle=0  RotationArbitraryAxis=[0 0 1]  FollAlignAxisA=+X  BaseAlignAxisA=+Y  FollAlignAxisB=+Y  BaseAlignAxisB=+Z  RotationSequenceAxes=FollowerAxes  RotationSequence=XYX  RotationSequenceAngles=[0 0 0]  RotationSequenceAnglesUnits=deg  RotationMatrix=[1 0 0; 0 1 0; 0 0 1]
  Rigid Transform6 : sm_lib/Frames and Transforms/Rigid Transform  Commented=on  TranslationMethod=Cartesian  TranslationStandardOffset=0  TranslationLengthUnit=m  TranslationStandardAxis=+Z  TranslationCartesianOffset=[-175 211 0]  TranslationROffset=0  TranslationROffsetUnits=m  TranslationZOffset=0  TranslationZOffsetUnits=m  TranslationThetaOffset=0  TranslationThetaOffsetUnits=deg  RotationMethod=StandardAxis  RotationAngleUnits=deg  RotationStandardAxis=+Z  RotationAngle=-90  RotationArbitraryAxis=[0 0 1]  FollAlignAxisA=+X  BaseAlignAxisA=+Y  FollAlignAxisB=+Y  BaseAlignAxisB=+Z  RotationSequenceAxes=FollowerAxes  RotationSequence=XYX  RotationSequenceAngles=[0 0 0]  RotationSequenceAnglesUnits=deg  RotationMatrix=[1 0 0; 0 1 0; 0 0 1]
  Rigid Transform7 : sm_lib/Frames and Transforms/Rigid Transform  Commented=on  TranslationMethod=Cartesian  TranslationStandardOffset=0  TranslationLengthUnit=m  TranslationStandardAxis=+Z  TranslationCartesianOffset=[-183 187 0]  TranslationROffset=0  TranslationROffsetUnits=m  TranslationZOffset=0  TranslationZOffsetUnits=m  TranslationThetaOffset=0  TranslationThetaOffsetUnits=deg  RotationMethod=StandardAxis  RotationAngleUnits=deg  RotationStandardAxis=+Z  RotationAngle=-90.0  RotationArbitraryAxis=[0 0 1]  FollAlignAxisA=+X  BaseAlignAxisA=+Y  FollAlignAxisB=+Y  BaseAlignAxisB=+Z  RotationSequenceAxes=FollowerAxes  RotationSequence=XYX  RotationSequenceAngles=[0 0 0]  RotationSequenceAnglesUnits=deg  RotationMatrix=[1 0 0; 0 1 0; 0 0 1]
  Rigid Transform8 : sm_lib/Frames and Transforms/Rigid Transform  Commented=on  TranslationMethod=Cartesian  TranslationStandardOffset=0  TranslationLengthUnit=m  TranslationStandardAxis=+Z  TranslationCartesianOffset=[-140 -250 0]  TranslationROffset=0  TranslationROffsetUnits=m  TranslationZOffset=0  TranslationZOffsetUnits=m  TranslationThetaOffset=0  TranslationThetaOffsetUnits=deg  RotationMethod=StandardAxis  RotationAngleUnits=deg  RotationStandardAxis=+Z  RotationAngle=0  RotationArbitraryAxis=[0 0 1]  FollAlignAxisA=+X  BaseAlignAxisA=+Y  FollAlignAxisB=+Y  BaseAlignAxisB=+Z  RotationSequenceAxes=FollowerAxes  RotationSequence=XYX  RotationSequenceAngles=[0 0 0]  RotationSequenceAnglesUnits=deg  RotationMatrix=[1 0 0; 0 1 0; 0 0 1]
  Rigid Transform9 : sm_lib/Frames and Transforms/Rigid Transform  Commented=on  TranslationMethod=Cartesian  TranslationStandardOffset=0  TranslationLengthUnit=m  TranslationStandardAxis=+Z  TranslationCartesianOffset=[-155 -250 0]  TranslationROffset=0  TranslationROffsetUnits=m  TranslationZOffset=0  TranslationZOffsetUnits=m  TranslationThetaOffset=0  TranslationThetaOffsetUnits=deg  RotationMethod=StandardAxis  RotationAngleUnits=deg  RotationStandardAxis=+Z  RotationAngle=0  RotationArbitraryAxis=[0 0 1]  FollAlignAxisA=+X  BaseAlignAxisA=+Y  FollAlignAxisB=+Y  BaseAlignAxisB=+Z  RotationSequenceAxes=FollowerAxes  RotationSequence=XYX  RotationSequenceAngles=[0 0 0]  RotationSequenceAnglesUnits=deg  RotationMatrix=[1 0 0; 0 1 0; 0 0 1]
  Simscape Bus : SimscapeBus  HierarchyStrings=Terreno
  Sweet&Coffee : sm_lib/Body Elements/File Solid  Commented=on  ExtGeomFileName=Edificios\sweet.stl  UnitType=Custom  ExtGeomFileUnits=m  StepReaderType=HEX  ExportConvexHullGeometry=off  InertiaType=PointMass  Mass=100  MassUnits=kg  CenterOfMass=[0 0 0]  CenterOfMassUnits=m  MomentsOfInertia=[1 1 1]  MomentsOfInertiaUnits=kg*m^2  ProductsOfInertia=[0 0 0]  ProductsOfInertiaUnits=kg*m^2  BasedOnType=DensityFromFile  Density=1000  DensityUnits=kg/m^3  DoExposeReferenceFrame=on  SerializedFrames=<Frames/>  GraphicType=FromGeometry  MarkerShape=Sphere  MarkerSize=10  GraphicVisPropType=SimpleVisualProperties  GraphicDiffuseColor=[0.0 0.4 0.2]  GraphicSpecularColor=[0.5 0.5 0.5 1.0]  GraphicAmbientColor=[0.15 0.15 0.15 1.0]  GraphicEmissiveColor=[0.0 0.0 0.0 1.0]  GraphicShininess=75  GraphicOpacity=1.0
  copias : sm_lib/Body Elements/File Solid  Commented=on  ExtGeomFileName=Edificios\Copiadora.stl  UnitType=Custom  ExtGeomFileUnits=m  StepReaderType=HEX  ExportConvexHullGeometry=off  InertiaType=PointMass  Mass=1000  MassUnits=kg  CenterOfMass=[0 0 0]  CenterOfMassUnits=m  MomentsOfInertia=[1 1 1]  MomentsOfInertiaUnits=kg*m^2  ProductsOfInertia=[0 0 0]  ProductsOfInertiaUnits=kg*m^2  BasedOnType=DensityFromFile  Density=1000  DensityUnits=kg/m^3  DoExposeReferenceFrame=on  SerializedFrames=<Frames/>  GraphicType=FromGeometry  MarkerShape=Sphere  MarkerSize=10  GraphicVisPropType=SimpleVisualProperties  GraphicDiffuseColor=[0.0 0.8 0.8]  GraphicSpecularColor=[0.5 0.5 0.5 1.0]  GraphicAmbientColor=[0.15 0.15 0.15 1.0]  GraphicEmissiveColor=[0.0 0.0 0.0 1.0]  GraphicShininess=75  GraphicOpacity=1.0
  planos : Subsystem
      settings: PortSchema="{\"entries\":[{\"content\":{\"sides\":[{\"content\":{\"connectorIds\":[]},\"type\":\"ConnectorPlacement.EquallySpacedRectSide\",\"uuid\":\"8da2d51d-cb04-40fd-b9e8-96e8eb5e3ca0\"},{\"content\":{\"connectorIds\":[\"RConn1\"],\"side\":\"RIGHT\"},\"type\":\"ConnectorPlacement.EquallySpacedRectSide\",\"uuid\":\"5658307d-c027-4fc3-a114-17c88b2e5db8\"},{\"content\":{\"connectorIds\":[],\"side\":\"TOP\"},\"type\":\"ConnectorPlacement.EquallySpacedRectSide\",\"uuid\":\"dfebcf2d-7098-4df6-aedf-48312a55bd34\"},{\"content\":{\"connectorIds\":[\"RConn2\"],\"side\":\"BOTTOM\"},\"type\":\"ConnectorPlacement.EquallySpacedRectSide\",\"uuid\":\"b261f848-4da2-49ad-8ec5-afbba00f5667\"}]},\"type\":\"ConnectorPlacement.EquallySpacedConnector\",\"uuid\":\"2edc3760-4540-4e03-af7a-55d7817fba59\"}],\"packageUris\":[\"http://schema.mathworks.com/mf0/Connector/R2020b\"],\"version\":\"1.0\"}"
  rampas : Subsystem
      settings: PortSchema="{\"entries\":[{\"content\":{\"sides\":[{\"content\":{\"connectorIds\":[]},\"type\":\"ConnectorPlacement.EquallySpacedRectSide\",\"uuid\":\"2296deee-340d-4a27-80fd-f37d09d83e3e\"},{\"content\":{\"connectorIds\":[\"RConn1\"],\"side\":\"RIGHT\"},\"type\":\"ConnectorPlacement.EquallySpacedRectSide\",\"uuid\":\"a80c974c-2473-4cac-9d69-af15faf658c6\"},{\"content\":{\"connectorIds\":[\"LConn1\"],\"side\":\"TOP\"},\"type\":\"ConnectorPlacement.EquallySpacedRectSide\",\"uuid\":\"5ae9daad-0b69-44eb-89df-542b4c4606cf\"}]},\"type\":\"ConnectorPlacement.EquallySpacedConnector\",\"uuid\":\"80df94f8-cd7c-4688-8ea4-a73f52f8abd9\"}],\"packageUris\":[\"http://schema.mathworks.com/mf0/Connector/R2020b\"],\"version\":\"1.0\"}"
  Conn3 : PMIOPort  Side=Left
  Z : PMIOPort  Port=2  Side=Right
  connections:
  Sweet&Coffee/RConn1 -- Rigid Transform1/LConn1
  copias/RConn1 -- Rigid Transform2/LConn1
  Fiec Nueva/RConn1 -- Rigid Transform4/LConn1
  Rigid Transform7/LConn1 -- Fiec Vieja2/RConn1
  Rigid Transform6/LConn1 -- Fiec Vieja1/RConn1
  Oficinas FIEC/RConn1 -- Rigid Transform8/LConn1
  Aulas FIMCP/RConn1 -- Rigid Transform9/LConn1
  Rigid Transform10/LConn1 -- Patio de comidas/RConn1
  DecanatoFIMCP/RConn1 -- Rigid Transform11/LConn1
  Aulas FICT/RConn1 -- Rigid Transform12/LConn1
  Rigid Transform13/LConn1 -- Fiec Lab y Fiec Vieja/RConn1
  FCNM/RConn1 -- Rigid Transform14/LConn1
  Rigid Transform11/RConn1 -- rampas/LConn1 -- planos/RConn2 -- Floor/LConn1 -- Rigid Transform5/RConn1 -- Rigid Transform14/RConn1 -- Rigid Transform1/RConn1 -- Conn3/RConn1 -- Rigid Transform8/RConn1 -- Rigid Transform13/RConn1 -- Rigid Transform7/RConn1 -- Rigid Transform6/RConn1 -- Rigid Transform12/RConn1 -- Rigid Transform3/RConn1 -- Rigid Transform4/RConn1 -- Rigid Transform2/RConn1 -- Rigid Transform9/RConn1 -- Rigid Transform10/RConn1
  File Solid/RConn1 -- Rigid Transform3/LConn1
  Z/RConn1 -- rampas/RConn1 -- planos/RConn1 -- Simscape Bus/RConn1
  Floor/RConn1 -- Simscape Bus/LConn1
  File Solid1/RConn1 -- Rigid Transform5/LConn1
